simulink model "cdr_model"  (R2020a)
settings: Solver=FixedStepAuto  StartTime=0.0  StopTime=100  FixedStep=1e-3  MaxStep=1e-5  RelTol=1e-3
libraries: dspsigops x4
settings Model: Creator=hassa  LastModifiedBy=hassa

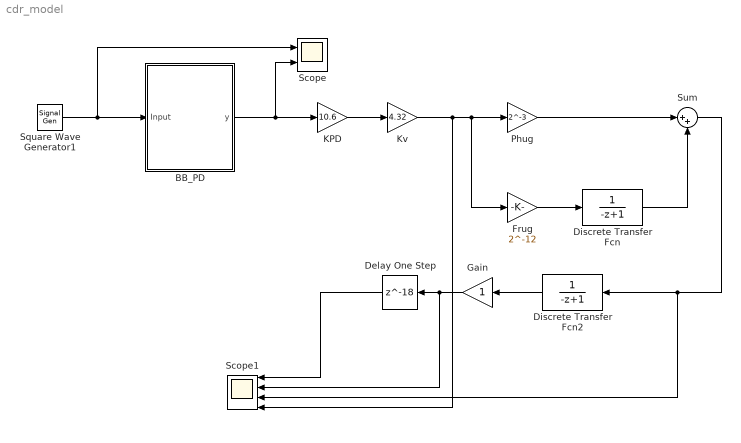
== system cdr_model ==
  BB_PD : Subsystem
  Delay One Step : Delay  DelayLength=18
  Discrete Transfer Fcn : DiscreteTransferFcn  Denominator=[-1 1]
  Discrete Transfer Fcn2 : DiscreteTransferFcn  Denominator=[-1 1]
  Frug : Gain  Gain=2^-12
  Gain : Gain
  KPD : Gain  Gain=10.6
  Kv : Gain  Gain=4.32
  Phug : Gain  Gain=2^-3
  Scope : Scope  NumInputPorts=2
  Scope1 : Scope  NumInputPorts=4
  Square Wave Generator1 : SignalGenerator  WaveForm=square  Frequency=2*pi*50  Units=rad/sec
  Sum : Sum  Inputs=|++
  wires:
  Square Wave Generator1/1 -> Scope/1, BB_PD/1(Input)
  BB_PD/1(y) -> KPD/1, Scope/2
  KPD/1 -> Kv/1
  Kv/1 -> Scope1/4, Frug/1, Phug/1
  Frug/1 -> Discrete Transfer Fcn/1
  Phug/1 -> Sum/1
  Discrete Transfer Fcn/1 -> Sum/2
  Sum/1 -> Scope1/3, Discrete Transfer Fcn2/1
  Discrete Transfer Fcn2/1 -> Gain/1
  Gain/1 -> Scope1/2, Delay One Step/1
  Delay One Step/1 -> Scope1/1

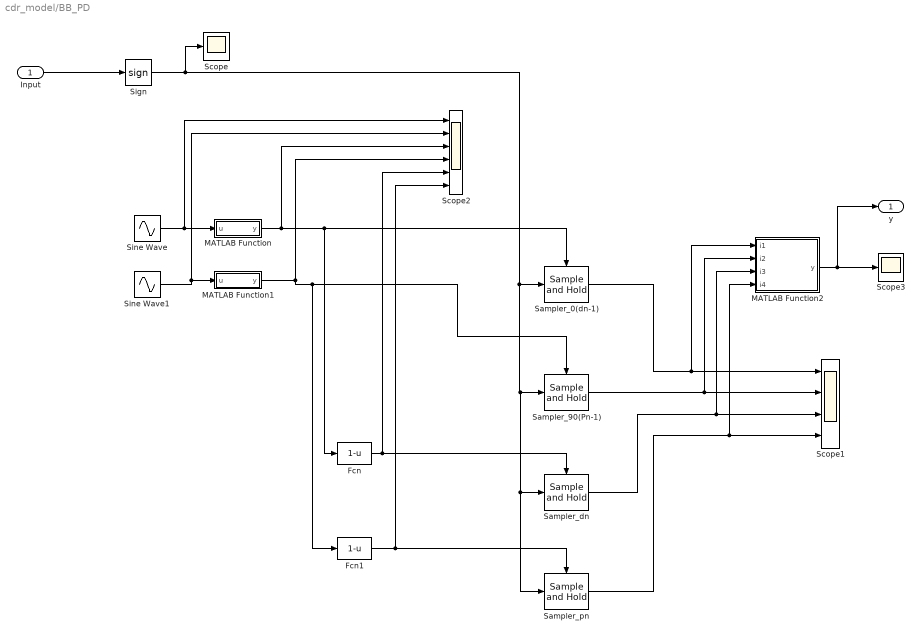
== system cdr_model/BB_PD ==
  Input : Inport
  Fcn : Fcn  Expr=1-u
  Fcn1 : Fcn  Expr=1-u
  MATLAB Function : MATLAB Function  TreatAsAtomicUnit=on
  MATLAB Function1 : MATLAB Function  TreatAsAtomicUnit=on
  MATLAB Function2 : MATLAB Function  TreatAsAtomicUnit=on
  Sampler_0(dn-1) : dspsigops/Sample and Hold  trig=Rising edge  initCond=0  latchinput=off
  Sampler_90(Pn-1) : dspsigops/Sample and Hold  trig=Rising edge  initCond=0  latchinput=off
  Sampler_dn : dspsigops/Sample and Hold  trig=Rising edge  initCond=0  latchinput=off
  Sampler_pn : dspsigops/Sample and Hold  trig=Rising edge  initCond=0  latchinput=off
  Scope : Scope
  Scope1 : Scope  NumInputPorts=4
  Scope2 : Scope  NumInputPorts=6
  Scope3 : Scope
  Sign : Signum
  Sine Wave : Sin  Frequency=2*pi*50  SampleTime=0
  Sine Wave1 : Sin  Frequency=2*pi*50  Phase=-pi/2  SampleTime=0
  y : Outport
  wires:
  MATLAB Function1/1(y) -> Fcn1/1, Sampler_90(Pn-1)/Trigger, Scope2/4
  Sine Wave/1 -> Scope2/1, MATLAB Function/1(u)
  Sampler_pn/1 -> MATLAB Function2/4(i4), Scope1/4
  MATLAB Function/1(y) -> Scope2/3, Sampler_0(dn-1)/Trigger, Fcn/1
  Sign/1 -> Sampler_pn/1, Sampler_dn/1, Sampler_90(Pn-1)/1, Sampler_0(dn-1)/1, Scope/1
  Sampler_0(dn-1)/1 -> MATLAB Function2/1(i1), Scope1/1
  Sine Wave1/1 -> MATLAB Function1/1(u), Scope2/2
  Sampler_90(Pn-1)/1 -> MATLAB Function2/2(i2), Scope1/2
  Sampler_dn/1 -> MATLAB Function2/3(i3), Scope1/3
  Fcn1/1 -> Sampler_pn/Trigger, Scope2/6
  Fcn/1 -> Sampler_dn/Trigger, Scope2/5
  Input/1 -> Sign/1
  MATLAB Function2/1(y) -> y/1, Scope3/1

== matlab function cdr_model/BB_PD/MATLAB Function1 ==
  data: u input; y output
function y = fcn(u)
threshold = 0;

if u > threshold
y = 1;
else 
y = 0

end

== matlab function cdr_model/BB_PD/MATLAB Function ==
  data: u input; y output
function y = fcn(u)
threshold = 0;

if u > threshold
y = 1;
else 
y = 0

end

== matlab function cdr_model/BB_PD/MATLAB Function2 ==
  data: i1 input; i2 input; i3 input; i4 input; y output
function y = fcn(i1, i2, i3, i4)

u1 = (i1==i2);
u2 = (i3==i4);

if u1 && u2
    y = 0;   %No Transition
elseif u1
    y = 1;   %early
elseif u2
    y = 2;   %late
else
    y = 0;   %No Transition
end    

disp(y)
end
